simulink model "MCC_retour_etat_estime_Kal"  (R2024a)
settings: Solver=VariableStepAuto  StartTime=0.0  StopTime=Tfinal  FixedStep=1e-3  RelTol=1e-3
undefined symbols (not defined in the file): A, B_sim, C, C_kal, K_lqr, L_kal, Nbar, Tmec, x0
libraries: simulink x1
settings Model: Creator=DELL  LastModifiedBy=DELL
settings OptimizationCC: DefaultParameterBehavior=Inlined  EnhancedBackFolding=on  PassReuseOutputArgsAs=Individual arguments  OptimizeBlockOrder=speed  DifferentSizesBufferReuse=on  OptimizationCustomize=off  EfficientTunableParamExpr=on
settings DebuggingCC: ParameterTunabilityLossMsg=error
settings SFSimCC: MATLABDynamicMemAlloc=off
settings RTWCC: Description=Create Visual C/C++ Solution File for Embedded Coder  SystemTargetFile=ert.tlc  TemplateMakefile=RTW.MSVCBuild  GenerateReport=on  LaunchReport=on
settings CodeAppCC: ForceParamTrailComments=on  IgnoreCustomStorageClasses=off  OperatorAnnotations=on  SimulinkDataObjDesc=on  SFDataObjDesc=on  InsertBlockDesc=on
settings ERTTargetCC: TargetLangStandard=C99 (ISO)  GenerateSampleERTMain=on  CodeInterfacePackaging=Reusable function  SupportContinuousTime=on  InlinedParameterPlacement=NonHierarchical  ERTCustomFileTemplate=example_file_process.tlc

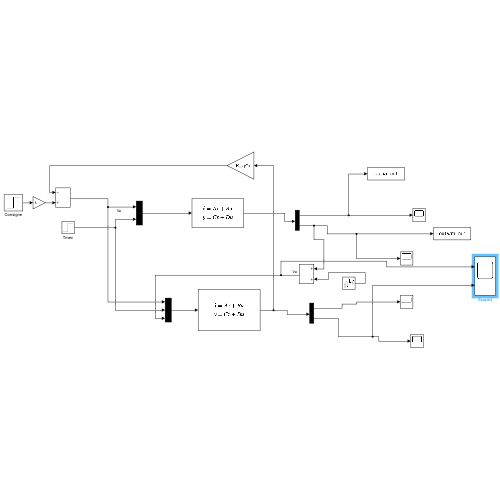
[thumbnail: Simulink's stored preview of the top-level diagram]
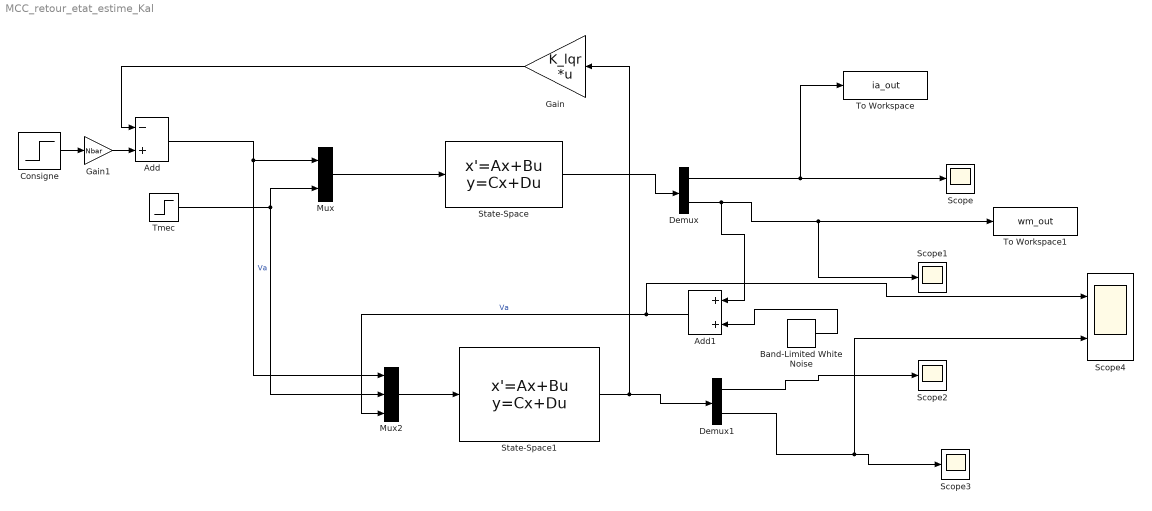
== system MCC_retour_etat_estime_Kal ==
  Add : Sum  Inputs=-+
  Add1 : Sum
  Band-Limited White Noise : simulink/Sources/Band-Limited White Noise  Cov=10  Ts=0.001  seed=[23341]
  Consigne : Step  Time=0  After=100  SampleTime=0
  Demux : Demux  Outputs=2
  Demux1 : Demux  Outputs=2
  Gain : Gain  Gain=K_lqr  Multiplication=Matrix(K*u)
  Gain1 : Gain  Gain=Nbar
  Mux : Mux  Inputs=2
  Mux2 : Mux  Inputs=3
  Scope{,1..3} (4 alike) : Scope
  Scope4 : Scope  NumInputPorts=2
  State-Space : StateSpace  A=A  B=B_sim  C=C  D=zeros(2,2)  InitialCondition=x0
  State-Space1 : StateSpace  A=A - L_kal * C_kal  B=[B_sim, L_kal]  C=eye(2)  D=zeros(2, 3)  InitialCondition=x0
  Tmec : Step  Time=0.5  After=Tmec  SampleTime=0
  To Workspace : ToWorkspace  VariableName=ia_out  SaveFormat=Timeseries  SampleTime=-1
  To Workspace1 : ToWorkspace  VariableName=wm_out  SaveFormat=Timeseries  SampleTime=-1
  wires:
  Mux/1 -> State-Space/1
  Tmec/1 -> Mux2/2, Mux/2
  Demux/1 -> Scope/1, To Workspace/1
  Gain/1 -> Add/1
  State-Space/1 -> Demux/1
  Mux2/1 -> State-Space1/1
  State-Space1/1 -> Gain/1, Demux1/1
  Demux1/1 -> Scope2/1
  Demux1/2 -> Scope4/2, Scope3/1
  Add/1 -> Mux2/1, Mux/1  "Va"
  Consigne/1 -> Gain1/1
  Demux/2 -> Add1/1, Scope1/1, To Workspace1/1
  Gain1/1 -> Add/2
  Add1/1 -> Scope4/1, Mux2/3  "Va"
  Band-Limited White Noise/1 -> Add1/2
